simulink model "NeuroSama"  (R2024b)
settings: Solver=VariableStepAuto  StartTime=0.0  StopTime=25  RelTol=1e-3
libraries: simulink x2
settings Model: Creator=Dr.Red  LastModifiedBy=Dr.Red

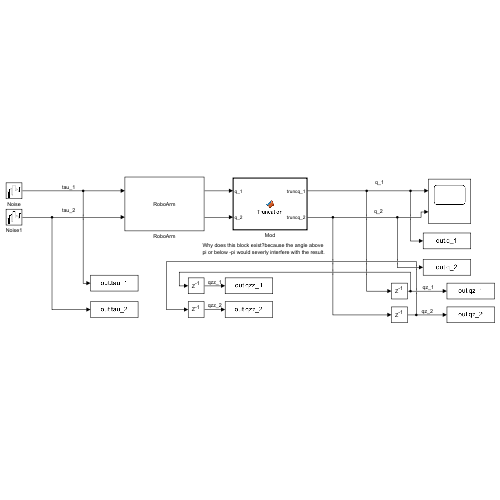
[thumbnail: Simulink's stored preview of the top-level diagram]
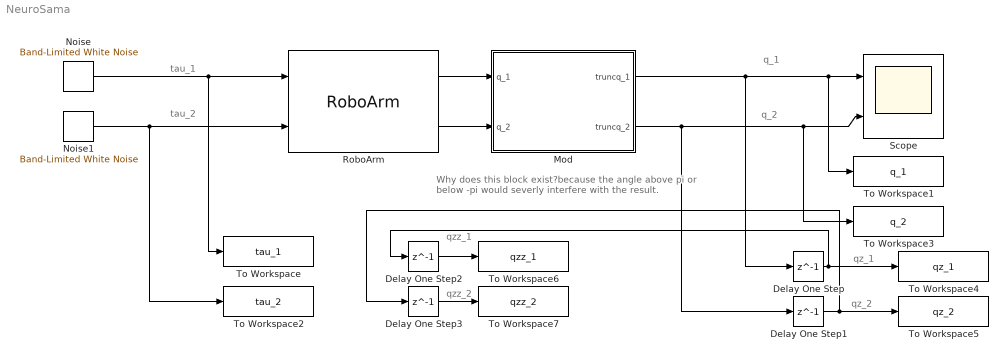
== system NeuroSama ==
  note: Why does this block exist?because the angle above
      | pi or below -pi would severly interfere with the result.
  note: tau_2
  note: tau_1
  note: q_2
  note: q_1
  note: qz_1
  note: qz_2
  note: qzz_1
  note: qzz_2
  Delay One Step{,1..3} (4 alike) : Delay  DelayLength=1
  Mod : MATLAB Function  TreatAsAtomicUnit=on
  Noise : simulink/Sources/Band-Limited White Noise  Cov=[0.003]  Ts=0.005  seed=[23340]
  Noise1 : simulink/Sources/Band-Limited White Noise  Cov=[0.003]  Ts=0.005  seed=[11451]
  RoboArm : M-S-Function  FunctionName=RoboArm  Parameters=0, 0, 0, 0
  Scope : Scope  NumInputPorts=2
  To Workspace : ToWorkspace  VariableName=tau_1  SampleTime=-1
  To Workspace1 : ToWorkspace  VariableName=q_1  SampleTime=-1
  To Workspace2 : ToWorkspace  VariableName=tau_2  SampleTime=-1
  To Workspace3 : ToWorkspace  VariableName=q_2  SampleTime=-1
  To Workspace4 : ToWorkspace  VariableName=qz_1  SampleTime=-1
  To Workspace5 : ToWorkspace  VariableName=qz_2  SampleTime=-1
  To Workspace6 : ToWorkspace  VariableName=qzz_1  SampleTime=-1
  To Workspace7 : ToWorkspace  VariableName=qzz_2  SampleTime=-1
  wires:
  Noise/1 -> To Workspace/1, RoboArm/1
  Noise1/1 -> To Workspace2/1, RoboArm/2
  Mod/1(truncq_1) -> Delay One Step/1, To Workspace1/1, Scope/1
  Mod/2(truncq_2) -> Scope/2, To Workspace3/1, Delay One Step1/1
  Delay One Step/1 -> To Workspace4/1, Delay One Step2/1
  Delay One Step1/1 -> To Workspace5/1, Delay One Step3/1
  Delay One Step2/1 -> To Workspace6/1
  Delay One Step3/1 -> To Workspace7/1
  RoboArm/1 -> Mod/1(q_1)
  RoboArm/2 -> Mod/2(q_2)

== matlab function NeuroSama/Mod ==
  data: q_1 input; truncq_1 output; q_2 input; truncq_2 output
function [truncq_1,truncq_2] = Truncation(q_1,q_2)

truncq_1 = mod( q_1 + pi, 2 * pi ) - pi;
truncq_2 = mod( q_2 + pi, 2 * pi ) - pi;
